simulink model "threepost_sim"  (R2020a)
settings: Solver=ode15s  StartTime=0.0  StopTime=T  FixedStep=0.00005  MaxStep=0.0005  RelTol=1e-3  EnableMultiTasking=on
values from neighbouring files (symbols this model uses):
  I_sat = [1/12*m_sat*(3*r^2+h^2),0,0;0,1/12*m_sat*(3*r^2+h^2),0;0,0,1/2*m_sat*r^2]    [berthing_sim_example_run.m]
  kd = 0.00005*[1;1;1;1;1;1;1]    [berthing_sim_example_run.m]
  ki = 0.001*ones(7,1)    [berthing_sim_example_run.m]
  kp = 5*[1;1;1;1;1;1;1]    [berthing_sim_example_run.m]
  m_sat = 2200    [berthing_sim_example_run.m]
  Pd = PBT0    [berthing_sim_example_run.m]
  q0 = [-0.0572;0.8617;0;-1.2870;0.0002;0.4292;0.0570]    [berthing_sim_example_run.m]
  qdot0 = zeros(7,1)    [berthing_sim_example_run.m]
  qlimit = [robot_const(1).limit.lower_joint_limit,     robot_const(1).limit.upper_joint_limit]    [berthing_sim_example_run.m]
  qm0 = robot_const.mprops.N.*q0    [berthing_sim_example_run.m]
  qmdot0 = zeros(7,1)    [berthing_sim_example_run.m]
  r = 0.7    [berthing_sim_example_run.m]
  ts_control = 0.002    [berthing_sim_example_run.m]
undefined symbols (not defined in the file or in its folder): robot_const, rot, X, Y, Z
libraries: sm_lib x58, nesl_utility x40, simulink x7
(part 1 of 3)
settings Model: Creator=Restore  LastModifiedBy=davidcarabis
settings SolverCC: MaxOrder=1  AutoInsertRateTranBlk=on
settings DataIOCC: ReturnWorkspaceOutputs=off
settings OptimizationCC: LifeSpan=inf
settings DebuggingCC: AllowSymbolicDim=off  SFUnexpectedBacktrackingDiag=warning  SFNoUnconditionalDefaultTransitionDiag=warning  SFExecutionAtInitializationDiag=none  ArithmeticOperatorsInVariantConditions=warning
settings SFSimCC: SimUseLocalCustomCode=off  CustomCodeUndefinedFunction=UseInterfaceOnly
settings RTWCC: RTWUseLocalCustomCode=off
settings CodeAppCC: StateflowObjectComments=on
settings GRTTargetCC: TargetLangStandard=C89/C90 (ANSI)
settings ConfigComp: CovMetricSettings=dw  CovHtmlReporting=on  CovSaveCumulativeToWorkspaceVar=on  CovSaveSingleToWorkspaceVar=on  CovExternalEMLEnable=off  CovSFcnEnable=off
settings SimscapeCC: SimscapeNominalValues="[{\"value\":\"10\",\"unit\":\"V\"},{\"value\":\"1\",\"unit\":\"A\"},{\"value\":\"10\",\"unit\":\"N*m\"},{\"value\":\"10\",\"unit\":\"bar\"},{\"value\":\"100\",\"unit\":\"kJ/kg\"},{\"value\":\"1\",\"unit\":\"kW\"},{\"value\":\"300\",\"unit\":\"K\"},{\"value\":\"100\",\"unit\":\"cm^3/s\"},{\"value\":\"1\",\"unit\":\"kN\"},{\"value\":\"1\",\"unit\":\"g/cm^3\"},{\"value\":\"1\",\"unit\":\"l\"},{\"value\":\"1\",\"unit\":\"cm^2\"},{\"value\":\"60\",\"unit\":\"Hz\"}]"  SimscapeLogType=all  SimscapeLogDataHistory=10000
settings ConfigurationSet: Description=SimMechanics 2G

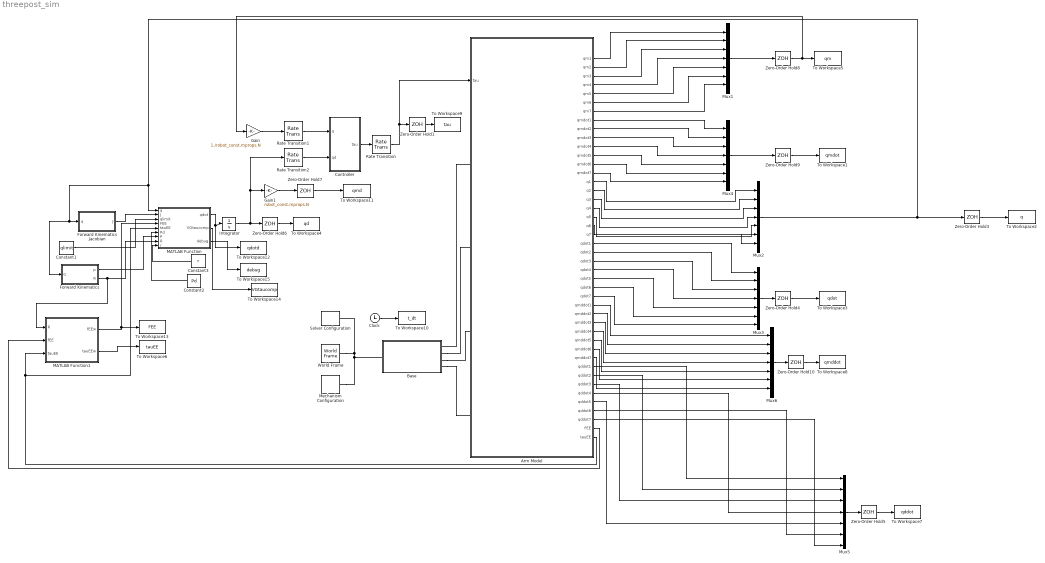
== system threepost_sim ==
  " Forward Kinematics Jacobian" : Subsystem  mask{H=robot_const(1).kin.H, P=robot_const.kin.P}
      mask prompts: H "Actuator Axes"; P "Actuator Displacements"
  Arm Model : Subsystem
  Base : Subsystem
  Clock : Clock
  Constant1 : Constant  Value=qlimit
  Constant2 : Constant  Value=Pd
  Constant3 : Constant  Value=r
  Controller : Subsystem
  Forward Kinematics : Subsystem  mask{H=robot_const(1).kin.H, P=robot_const(1).kin.P}
      mask prompts: H "Actuator Axes"; P "Actuator Displacements"
  Gain : Gain  Gain=1./robot_const.mprops.N
  Gain1 : Gain  Gain=robot_const.mprops.N
  Integrator : Integrator  InitialCondition=q0
  MATLAB Function : MATLAB Function  TreatAsAtomicUnit=on
  MATLAB Function1 : MATLAB Function  TreatAsAtomicUnit=on
  Mechanism Configuration : sm_lib/Utilities/Mechanism Configuration  UniformGravity=None  GravityVector=[0 0 -9.80665]  GravityUnits=m/s^2  LinearizationDelta=0.001
  Mux{1..6} (6 alike) : Mux  Inputs=7
  Rate Transition : RateTransition
  Rate Transition1 : RateTransition
  Rate Transition2 : RateTransition
  Solver Configuration : nesl_utility/Solver Configuration  PhysicalDomain=network_engine_domain  SubClassName=solver  LeftPortType=input  RightPortType=generic  Tones=[]  Harmonics=[]  SimulateNoise=off  Profile=off  UseLocalSampling=off  EnableSwitchedLinearOptims=on  FrequencyDomain=off  UseCCode=off  RelTol=0.001  AbsTol=1e-06  MinStep=1e-09  ToWorkspace=off  RevertToSquareIcSolve=off  NumHomotopyIterations=100  PhasorMode=off  PhasorModeNumHarmonics=1  DoDC=off  ResidualTolerance=1e-09  UseLocalSolver=off  LocalSolverChoice=NE_BACKWARD_EULER_ADVANCER  LocalSolverSampleTime=0.001  DoFixedCost=off  MaxNonlinIter=3  MaxModeIter=2  LinearAlgebra=Sparse  EquationFormulation=NE_TIME_EF  DelaysMemoryBudget=1024  AutomaticFiltering=on  FilteringTimeConstant=0.001  PartitionStorageMethod=AS_NEEDED  PartitionMemoryBudget=1024  PartitionMethod=FAST
  To Workspace1 : ToWorkspace  VariableName=qmdot  SampleTime=ts_control
  To Workspace10 : ToWorkspace  VariableName=t_dt  SampleTime=ts_control
  To Workspace11 : ToWorkspace  VariableName=qmd  SampleTime=-1
  To Workspace12 : ToWorkspace  VariableName=qdotd  SampleTime=-1
  To Workspace13 : ToWorkspace  VariableName=FEE  SampleTime=ts_control
  To Workspace14 : ToWorkspace  VariableName=VGtaucomp  SampleTime=-1
  To Workspace15 : ToWorkspace  VariableName=debug  SampleTime=-1
  To Workspace2 : ToWorkspace  VariableName=q  SampleTime=-1
  To Workspace3 : ToWorkspace  VariableName=qdot  SampleTime=-1
  To Workspace4 : ToWorkspace  VariableName=qd  SampleTime=-1
  To Workspace5 : ToWorkspace  VariableName=qm  SampleTime=ts_control
  To Workspace6 : ToWorkspace  VariableName=tauEE  SampleTime=ts_control
  To Workspace7 : ToWorkspace  VariableName=qddot  SampleTime=-1
  To Workspace8 : ToWorkspace  VariableName=qmddot  SampleTime=ts_control
  To Workspace9 : ToWorkspace  VariableName=tau  SampleTime=-1
  World Frame : sm_lib/Frames and Transforms/World Frame
  Zero-Order Hold{1,3..10} (9 alike) : ZeroOrderHold  SampleTime=ts_control
  wires:
  Arm Model/15(q1) -> Mux2/1
  Arm Model/16(q2) -> Mux2/2
  Arm Model/22(qdot1) -> Mux3/1
  Arm Model/23(qdot2) -> Mux3/2
  Mux3/1 -> Zero-Order Hold4/1
  Arm Model/17(q3) -> Mux2/3
  Arm Model/24(qdot3) -> Mux3/3
  Arm Model/18(q4) -> Mux2/4
  Arm Model/25(qdot4) -> Mux3/4
  Arm Model/19(q5) -> Mux2/5
  Arm Model/26(qdot5) -> Mux3/5
  Arm Model/20(q6) -> Mux2/6
  Arm Model/27(qdot6) -> Mux3/6
  Arm Model/21(q7) -> Mux2/7
  Arm Model/28(qdot7) -> Mux3/7
  Mux2/1 -> " Forward Kinematics Jacobian"/1(q), Forward Kinematics/1(q), MATLAB Function/1(q), Zero-Order Hold3/1
  Arm Model/36(qddot1) -> Mux5/1
  Arm Model/37(qddot2) -> Mux5/2
  Arm Model/38(qddot3) -> Mux5/3
  Mux5/1 -> Zero-Order Hold5/1
  Arm Model/39(qddot4) -> Mux5/4
  Arm Model/40(qddot5) -> Mux5/5
  Arm Model/41(qddot6) -> Mux5/6
  Arm Model/42(qddot7) -> Mux5/7
  Integrator/1 -> Gain1/1, Rate Transition2/1, Zero-Order Hold6/1
  Clock/1 -> To Workspace10/1
  Zero-Order Hold3/1 -> To Workspace2/1
  Zero-Order Hold4/1 -> To Workspace3/1
  Zero-Order Hold5/1 -> To Workspace7/1
  Zero-Order Hold6/1 -> To Workspace4/1
  Arm Model/1(qm1) -> Mux1/1
  Arm Model/2(qm2) -> Mux1/2
  Arm Model/3(qm3) -> Mux1/3
  Arm Model/4(qm4) -> Mux1/4
  Arm Model/5(qm5) -> Mux1/5
  Arm Model/6(qm6) -> Mux1/6
  Arm Model/7(qm7) -> Mux1/7
  Arm Model/8(qmdot1) -> Mux4/1
  Arm Model/9(qmdot2) -> Mux4/2
  Arm Model/10(qmdot3) -> Mux4/3
  Arm Model/11(qmdot4) -> Mux4/4
  Arm Model/12(qmdot5) -> Mux4/5
  Arm Model/13(qmdot6) -> Mux4/6
  Arm Model/14(qmdot7) -> Mux4/7
  Arm Model/29(qmddot1) -> Mux6/1
  Arm Model/30(qmddot2) -> Mux6/2
  Arm Model/31(qmddot3) -> Mux6/3
  Arm Model/32(qmddot4) -> Mux6/4
  Arm Model/33(qmddot5) -> Mux6/5
  Arm Model/34(qmddot6) -> Mux6/6
  Arm Model/35(qmddot7) -> Mux6/7
  Mux1/1 -> Zero-Order Hold8/1
  Mux4/1 -> Zero-Order Hold9/1
  Mux6/1 -> Zero-Order Hold10/1
  Zero-Order Hold9/1 -> To Workspace1/1
  Zero-Order Hold10/1 -> To Workspace8/1
  Zero-Order Hold8/1 -> Gain/1, To Workspace5/1
  Controller/1(tau) -> Rate Transition/1
  Rate Transition1/1 -> Controller/1(q)
  Rate Transition2/1 -> Controller/2(qd)
  Zero-Order Hold1/1 -> To Workspace9/1
  Gain/1 -> Rate Transition1/1
  Gain1/1 -> Zero-Order Hold7/1
  Zero-Order Hold7/1 -> To Workspace11/1
  Rate Transition/1 -> Zero-Order Hold1/1, Arm Model/1(tau)
  MATLAB Function/1(qdot) -> To Workspace12/1, Integrator/1
  " Forward Kinematics Jacobian"/1(J) -> MATLAB Function/2(J)
  Constant1/1 -> MATLAB Function/3(qlimit)
  Constant2/1 -> MATLAB Function/6(Pd)
  Forward Kinematics/2(R) -> MATLAB Function1/1(R), MATLAB Function/8(R)
  Forward Kinematics/1(p) -> MATLAB Function/7(P)
  MATLAB Function1/2(tauEEw) -> To Workspace6/1
  MATLAB Function1/1(fEEw) -> MATLAB Function/4(FEE), To Workspace13/1
  Arm Model/43(FEE) -> MATLAB Function1/2(fEE)
  Arm Model/44(tauEE) -> MATLAB Function/5(tauEE), MATLAB Function1/3(tauEE)
  Constant3/1 -> MATLAB Function/9(r)
  MATLAB Function/2(VGtaucomp) -> To Workspace14/1
  MATLAB Function/3(debug) -> To Workspace15/1
  connections:
  Mechanism Configuration/RConn1 -- Solver Configuration/RConn1 -- World Frame/RConn1 -- Base/LConn1
  Arm Model/LConn1 -- Base/RConn1
  Base/RConn2 -- Arm Model/LConn2
  Base/RConn3 -- Arm Model/LConn3
  Base/RConn4 -- Arm Model/LConn4

== system threepost_sim/ Forward Kinematics Jacobian ==
  q : Inport
  Forward Kinematics Jacobian : MATLAB Function  TreatAsAtomicUnit=on
  J : Outport
  wires:
  q/1 -> Forward Kinematics Jacobian/1(q)
  Forward Kinematics Jacobian/1(J) -> J/1

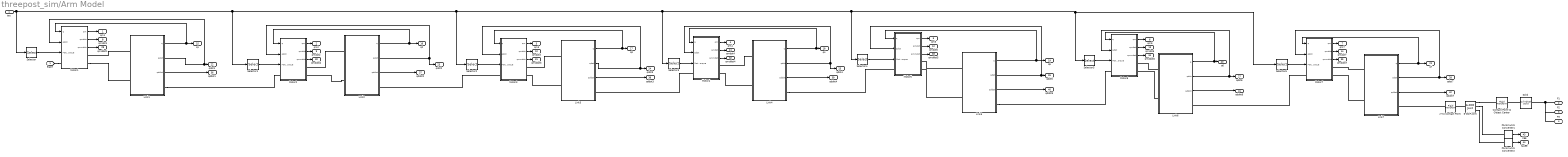
== system threepost_sim/Arm Model ==
  tau : Inport
  6-DOF Joint : sm_lib/Joints/6-DOF Joint  JointMode=Normal  SenseConstraintForce=off  SenseConstraintForceX=off  SenseConstraintForceY=off  SenseConstraintForceZ=off  SenseConstraintTorque=off  SenseConstraintTorqueX=off  SenseConstraintTorqueY=off  SenseConstraintTorqueZ=off  SenseTotalForce=on  SenseTotalForceX=off  SenseTotalForceY=off  SenseTotalForceZ=off  SenseTotalTorque=on  SenseTotalTorqueX=off  SenseTotalTorqueY=off  SenseTotalTorqueZ=off  CompositeWrenchDir=BaseOnFollower  CompositeWrenchFrame=BaseFrame  PxEquilibriumPosition=0  PxEquilibriumPositionUnits=m  PxSpringStiffness=kt_contact  PxSpringStiffnessUnits=N/m  PxDampingCoefficient=bt_contact  PxDampingCoefficientUnits=N/(m/s)  PxTorqueActuationMode=NoTorque  PxMotionActuationMode=ComputedMotion  PxSensePosition=off  PxSenseVelocity=off  PxSenseAcceleration=off  PxSenseTorqueForce=off  PxSenseLowerLimitTorqueForce=off  PxSenseUpperLimitTorqueForce=off  PxLowerLimitSpecify=off  PxLowerLimitBound=-1  PxLowerLimitBoundUnits=m  PxLowerLimitStiffness=1e6  PxLowerLimitStiffnessUnits=N/m  PxLowerLimitDamping=1e3  PxLowerLimitDampingUnits=N/(m/s)  PxLowerLimitTransitionRegionWidth=1e-4  PxLowerLimitTransitionRegionWidthUnits=m  PxUpperLimitSpecify=off  PxUpperLimitBound=1  PxUpperLimitBoundUnits=m  PxUpperLimitStiffness=1e6  PxUpperLimitStiffnessUnits=N/m  PxUpperLimitDamping=1e3  PxUpperLimitDampingUnits=N/(m/s)  PxUpperLimitTransitionRegionWidth=1e-4  PxUpperLimitTransitionRegionWidthUnits=m  PxPositionTargetSpecify=on  PxPositionTargetPriority=High  PxPositionTargetValue=0  PxPositionTargetValueUnits=m  PxVelocityTargetSpecify=on  PxVelocityTargetPriority=High  PxVelocityTargetValue=0  PxVelocityTargetValueUnits=m/s  PyEquilibriumPosition=0  PyEquilibriumPositionUnits=m  PySpringStiffness=kt_contact  PySpringStiffnessUnits=N/m  PyDampingCoefficient=bt_contact  PyDampingCoefficientUnits=N/(m/s)  PyTorqueActuationMode=NoTorque  PyMotionActuationMode=ComputedMotion  PySensePosition=off  PySenseVelocity=off  PySenseAcceleration=off  PySenseTorqueForce=off  PySenseLowerLimitTorqueForce=off  PySenseUpperLimitTorqueForce=off  PyLowerLimitSpecify=off  PyLowerLimitBound=-1  PyLowerLimitBoundUnits=m  PyLowerLimitStiffness=1e6  PyLowerLimitStiffnessUnits=N/m  PyLowerLimitDamping=1e3  PyLowerLimitDampingUnits=N/(m/s)  PyLowerLimitTransitionRegionWidth=1e-4  PyLowerLimitTransitionRegionWidthUnits=m  PyUpperLimitSpecify=off  PyUpperLimitBound=1  PyUpperLimitBoundUnits=m  PyUpperLimitStiffness=1e6  PyUpperLimitStiffnessUnits=N/m  PyUpperLimitDamping=1e3  PyUpperLimitDampingUnits=N/(m/s)  PyUpperLimitTransitionRegionWidth=1e-4  PyUpperLimitTransitionRegionWidthUnits=m  PyPositionTargetSpecify=on  PyPositionTargetPriority=High  PyPositionTargetValue=0  PyPositionTargetValueUnits=m  PyVelocityTargetSpecify=on  PyVelocityTargetPriority=High  PyVelocityTargetValue=0  PyVelocityTargetValueUnits=m/s  PzEquilibriumPosition=0  PzEquilibriumPositionUnits=m  PzSpringStiffness=kt_contact  PzSpringStiffnessUnits=N/m  PzDampingCoefficient=bt_contact  PzDampingCoefficientUnits=N/(m/s)  PzTorqueActuationMode=NoTorque  PzMotionActuationMode=ComputedMotion  PzSensePosition=off  PzSenseVelocity=off  PzSenseAcceleration=off  PzSenseTorqueForce=off  PzSenseLowerLimitTorqueForce=off  PzSenseUpperLimitTorqueForce=off  PzLowerLimitSpecify=off  PzLowerLimitBound=-1  PzLowerLimitBoundUnits=m  PzLowerLimitStiffness=1e6  PzLowerLimitStiffnessUnits=N/m  PzLowerLimitDamping=1e3  PzLowerLimitDampingUnits=N/(m/s)  PzLowerLimitTransitionRegionWidth=1e-4  PzLowerLimitTransitionRegionWidthUnits=m  PzUpperLimitSpecify=off  PzUpperLimitBound=1  PzUpperLimitBoundUnits=m  PzUpperLimitStiffness=1e6  PzUpperLimitStiffnessUnits=N/m  PzUpperLimitDamping=1e3  PzUpperLimitDampingUnits=N/(m/s)  PzUpperLimitTransitionRegionWidth=1e-4  PzUpperLimitTransitionRegionWidthUnits=m  PzPositionTargetSpecify=on  PzPositionTargetPriority=High  PzPositionTargetValue=0  PzPositionTargetValueUnits=m  PzVelocityTargetSpecify=on  PzVelocityTargetPriority=High  PzVelocityTargetValue=0  PzVelocityTargetValueUnits=m/s  SphDefPosRotationMethod=None  SphDefPosRotationAngleUnits=deg  SphDefPosRotationStandardAxis=+Z  SphDefPosRotationAngle=0.0  SphDefPosRotationArbitraryAxis=[0 0 1]  SphDefPosFollAlignAxisA=+X  SphDefPosBaseAlignAxisA=+Y  SphDefPosFollAlignAxisB=+Y  SphDefPosBaseAlignAxisB=+Z  SphDefPosRotationSequenceAxes=FollowerAxes  SphDefPosRotationSequence=XYX  SphDefPosRotationSequenceAngles=[0 0 0]  SphDefPosRotationSequenceAnglesUnits=deg  SphDefPosRotationMatrix=[1 0 0; 0 1 0; 0 0 1]  SphEqPosRotationMethod=RotationMatrix  SphEqPosRotationAngleUnits=deg  SphEqPosRotationStandardAxis=+Z  SphEqPosRotationAngle=0.0  SphEqPosRotationArbitraryAxis=[0 0 1]  SphEqPosFollAlignAxisA=+X  SphEqPosBaseAlignAxisA=+Y  SphEqPosFollAlignAxisB=+Y  SphEqPosBaseAlignAxisB=+Z  SphEqPosRotationSequenceAxes=FollowerAxes  SphEqPosRotationSequence=XYX  SphEqPosRotationSequenceAngles=[0 0 0]  SphEqPosRotationSequenceAnglesUnits=deg  SphEqPosRotationMatrix=[1 0 0; 0 1 0; 0 0 1]  SphSpringStiffness=kr_contact  SphSpringStiffnessUnits=N*m/rad  SphDampingCoefficient=br_contact  SphDampingCoefficientUnits=N*m/(rad/s)  SphActuateTorqueX=off  SphActuateTorqueY=off  SphActuateTorqueZ=off  SphActuateTorque=off  SphTorqueActuationMode=NoTorque  SphMotionActuationMode=ComputedMotion  SphActuationFrame=BaseFrame  SphSensePosition=off  SphSenseVelocityX=off  SphSenseVelocityY=off  SphSenseVelocityZ=off  SphSenseVelocity=off  SphSenseAccelerationX=off  SphSenseAccelerationY=off  SphSenseAccelerationZ=off  SphSenseAcceleration=off  SphSenseTorqueX=off  SphSenseTorqueY=off  SphSenseTorqueZ=off  SphSenseTorqueForce=off  SphSenseLowerLimitTorqueMag=off  SphSenseUpperLimitTorqueMag=off  SphSensingFrame=BaseFrame  SphLowerLimitSpecify=off  SphLowerLimitBound=15  SphLowerLimitBoundUnits=deg  SphLowerLimitStiffness=1e4  SphLowerLimitStiffnessUnits=N*m/deg  SphLowerLimitDamping=10  SphLowerLimitDampingUnits=N*m/(deg/s)  SphLowerLimitTransitionRegionWidth=0.1  SphLowerLimitTransitionRegionWidthUnits=deg  SphUpperLimitSpecify=off  SphUpperLimitBound=45  SphUpperLimitBoundUnits=deg  SphUpperLimitStiffness=1e4  SphUpperLimitStiffnessUnits=N*m/deg  SphUpperLimitDamping=10  SphUpperLimitDampingUnits=N*m/(deg/s)  SphUpperLimitTransitionRegionWidth=0.1  SphUpperLimitTransitionRegionWidthUnits=deg  SphPositionTargetRotationMethod=RotationMatrix  SphPositionTargetRotationAngleUnits=deg  SphPositionTargetRotationStandardAxis=+Z  SphPositionTargetRotationAngle=0.0  SphPositionTargetRotationArbitraryAxis=[0 0 1]  SphPositionTargetFollAlignAxisA=+X  SphPositionTargetBaseAlignAxisA=+Y  SphPositionTargetFollAlignAxisB=+Y  SphPositionTargetBaseAlignAxisB=+Z  SphPositionTargetRotationSequenceAxes=FollowerAxes  SphPositionTargetRotationSequence=XYX  SphPositionTargetRotationSequenceAngles=[0 0 0]  SphPositionTargetRotationSequenceAnglesUnits=deg  SphPositionTargetRotationMatrix=[1 0 0; 0 1 0; 0 0 1]  SphPositionTargetSpecify=on  SphPositionTargetPriority=High  SphVelocityTargetValue=[0 0 0]  SphVelocityTargetValueUnits=deg/s  SphVelocityTargetSpecify=on  SphVelocityTargetPriority=High  SphVelocityTargetInFollowerFrame=on
  Contact Point to Object Center : sm_lib/Frames and Transforms/Rigid Transform  TranslationMethod=Cartesian  TranslationStandardOffset=0  TranslationLengthUnit=m  TranslationStandardAxis=+Z  TranslationCartesianOffset=PGsat  TranslationROffset=0  TranslationROffsetUnits=m  TranslationZOffset=0  TranslationZOffsetUnits=m  TranslationThetaOffset=0  TranslationThetaOffsetUnits=deg  RotationMethod=None  RotationAngleUnits=rad  RotationStandardAxis=+Z  RotationAngle=0  RotationArbitraryAxis=0  FollAlignAxisA=+X  BaseAlignAxisA=+Y  FollAlignAxisB=+Y  BaseAlignAxisB=+Z  RotationSequenceAxes=FollowerAxes  RotationSequence=XYX  RotationSequenceAngles=[0 0 0]  RotationSequenceAnglesUnits=deg  RotationMatrix=[1 0 0; 0 1 0; 0 0 1]
  J7 to Contact Point : sm_lib/Frames and Transforms/Rigid Transform  TranslationMethod=Cartesian  TranslationStandardOffset=0  TranslationLengthUnit=m  TranslationStandardAxis=+Z  TranslationCartesianOffset=robot_const.kin.P(:,8)  TranslationROffset=0  TranslationROffsetUnits=m  TranslationZOffset=0  TranslationZOffsetUnits=m  TranslationThetaOffset=0  TranslationThetaOffsetUnits=deg  RotationMethod=None  RotationAngleUnits=rad  RotationStandardAxis=+Z  RotationAngle=0  RotationArbitraryAxis=0  FollAlignAxisA=+X  BaseAlignAxisA=+Y  FollAlignAxisB=+Y  BaseAlignAxisB=+Z  RotationSequenceAxes=FollowerAxes  RotationSequence=XYX  RotationSequenceAngles=[0 0 0]  RotationSequenceAnglesUnits=deg  RotationMatrix=[1 0 0; 0 1 0; 0 0 1]
  Link1 : Subsystem  mask{q0=q0(1), qdot0=qdot0(1), r=0.1, l=0.27035, m=robot_const.mprops.m(1), I=robot_const.mprops.Ic(:,:,1), c=robot_const.mprops.c(:,1), p=[0;0;0.27035/2]}
      mask prompts: q0 "Initial Position (rad)"; qdot0 "Initial Speed (rad/s)"; r "Radius (m)"; l "Length (m)"; m "Mass (kg)"; I "Inertia Tensor (kg m^2)"; c "COG Vector (m)"; p "Link Frame Translation"
  Link2 : Subsystem  mask{q0=q0(2), qdot0=qdot0(2), r=0.1, l=0.2, m=robot_const.mprops.m(2), I=[1 0 0;0 0 1 ;0 1 0]*robot_const.mprops.Ic(:,:,2)*[1 0 0;0 0 1 ;0 1 0]', c=[1 0 0;0 0 1 ;0 1 0]*robot_const.mprops.c(:,2), p=[0;0;0]}
      mask prompts: q0 "Initial Position (rad)"; qdot0 "Initial Speed (rad/s)"; r "Radius (m)"; l "Length (m)"; m "Mass (kg)"; I "Inertia Tensor (kg m^2)"; c "COG Vector (m)"; p "Link Frame Translation"
  Link3 : Subsystem  mask{q0=q0(3), qdot0=qdot0(3), r=0.08, l=0.36435, m=robot_const.mprops.m(3), I=robot_const.mprops.Ic(:,:,3), c=robot_const.mprops.c(:,3), p=[0;0;0.36435/2]}
      mask prompts: q0 "Initial Position (rad)"; qdot0 "Initial Speed (rad/s)"; r "Radius (m)"; l "Length (m)"; m "Mass (kg)"; I "Inertia Tensor (kg m^2)"; c "COG Vector (m)"; p "Link Frame Translation"
  Link4 : Subsystem  mask{q0=q0(4), qdot0=qdot0(4), r=0.08, l=0.2, m=robot_const.mprops.m(4), I=[1 0 0;0 0 1 ;0 1 0]*robot_const.mprops.Ic(:,:,4)*[1 0 0;0 0 1 ;0 1 0]', c=[1 0 0;0 0 1 ;0 1 0]*robot_const.mprops.c(:,4), p=[0;0;0]}
      mask prompts: q0 "Initial Position (rad)"; qdot0 "Initial Speed (rad/s)"; r "Radius (m)"; l "Length (m)"; m "Mass (kg)"; I "Inertia Tensor (kg m^2)"; c "COG Vector (m)"; p "Link Frame Translation"
  Link5 : Subsystem  mask{q0=q0(5), qdot0=qdot0(5), r=0.08, l=0.37429, m=robot_const.mprops.m(5), I=robot_const.mprops.Ic(:,:,5), c=robot_const.mprops.c(:,5), p=[0;0;0.37429/2]}
      mask prompts: q0 "Initial Position (rad)"; qdot0 "Initial Speed (rad/s)"; r "Radius (m)"; l "Length (m)"; m "Mass (kg)"; I "Inertia Tensor (kg m^2)"; c "COG Vector (m)"; p "Link Frame Translation"
  Link6 : Subsystem  mask{q0=q0(6), qdot0=qdot0(6), r=0.08, l=0.2, m=robot_const.mprops.m(6), I=[1 0 0;0 0 1 ;0 1 0]*robot_const.mprops.Ic(:,:,6)*[1 0 0;0 0 1 ;0 1 0]', c=[1 0 0;0 0 1 ;0 1 0]*robot_const.mprops.c(:,6), p=[0;0;0]}
      mask prompts: q0 "Initial Position (rad)"; qdot0 "Initial Speed (rad/s)"; r "Radius (m)"; l "Length (m)"; m "Mass (kg)"; I "Inertia Tensor (kg m^2)"; c "COG Vector (m)"; p "Link Frame Translation"
  Link7 : Subsystem  mask{q0=q0(7), qdot0=qdot0(7), r=0.05, l=robot_const.kin.P(3,8), m=robot_const.mprops.m(7), I=robot_const.mprops.Ic(:,:,7), c=robot_const.mprops.c(:,7), p=robot_const.kin.P(:,8)/2}
      mask prompts: q0 "Initial Position (rad)"; qdot0 "Initial Speed (rad/s)"; r "Radius (m)"; l "Length (m)"; m "Mass (kg)"; I "Inertia Tensor (kg m^2)"; c "COG Vector (m)"; p "Link Frame Translation"
  Motor1 : Subsystem  mask{h=[1;0;0], alpha=0, p=[0;0;0], bm=robot_const.mprops.bm(1), Jm=robot_const.mprops.Im(1), N=robot_const.mprops.N(1), K=robot_const.mprops.K(1), bL=robot_const.mprops.bl(1), qm0=qm0(1), qmdot0=qmdot0(1)}
      mask prompts: h "Frame Rotation Axis"; alpha "Frame Rotation Angle (rad)"; p "Frame Translation (m)"; bm "Motor Friction"; Jm "Motor Inertia (kg m^2)"; N "Gear Ratio"; K "Spring Constant (Nm/rad)"; bL "Gearbox Friction (Nm s/rad)"; qm0 "Motor Initial Position"; qmdot0 "Motor Initial Velocity"
  Motor2 : Subsystem  mask{h=[1;0;0], alpha=-pi/2, p=robot_const.kin.P(:,2), bm=robot_const.mprops.bm(2), Jm=robot_const.mprops.Im(2), N=robot_const.mprops.N(2), K=robot_const.mprops.K(2), bL=robot_const.mprops.bl(2), qm0=qm0(2), qmdot0=qmdot0(2)}
      mask prompts: h "Frame Rotation Axis"; alpha "Frame Rotation Angle (rad)"; p "Frame Translation (m)"; bm "Motor Friction"; Jm "Motor Inertia (kg m^2)"; N "Gear Ratio"; K "Spring Constant (Nm/rad)"; bL "Gearbox Friction (Nm s/rad)"; qm0 "Motor Initial Position"; qmdot0 "Motor Initial Velocity"
  Motor3 : Subsystem  mask{h=[1;0;0], alpha=0, p=[0;0;0], bm=robot_const.mprops.bm(3), Jm=robot_const.mprops.Im(3), N=robot_const.mprops.N(3), K=robot_const.mprops.K(3), bL=robot_const.mprops.bl(3), qm0=qm0(3), qmdot0=qmdot0(3)}
      mask prompts: h "Frame Rotation Axis"; alpha "Frame Rotation Angle (rad)"; p "Frame Translation (m)"; bm "Motor Friction"; Jm "Motor Inertia (kg m^2)"; N "Gear Ratio"; K "Spring Constant (Nm/rad)"; bL "Gearbox Friction (Nm s/rad)"; qm0 "Motor Initial Position"; qmdot0 "Motor Initial Velocity"
  Motor4 : Subsystem  mask{h=[1;0;0], alpha=-pi/2, p=robot_const.kin.P(:,4), bm=robot_const.mprops.bm(4), Jm=robot_const.mprops.Im(4), N=robot_const.mprops.N(4), K=robot_const.mprops.K(4), bL=robot_const.mprops.bl(4), qm0=qm0(4), qmdot0=qmdot0(4)}
      mask prompts: h "Frame Rotation Axis"; alpha "Frame Rotation Angle (rad)"; p "Frame Translation (m)"; bm "Motor Friction"; Jm "Motor Inertia (kg m^2)"; N "Gear Ratio"; K "Spring Constant (Nm/rad)"; bL "Gearbox Friction (Nm s/rad)"; qm0 "Motor Initial Position"; qmdot0 "Motor Initial Velocity"
  Motor5 : Subsystem  mask{h=[1;0;0], alpha=0, p=[0;0;0], bm=robot_const.mprops.bm(5), Jm=robot_const.mprops.Im(5), N=robot_const.mprops.N(5), K=robot_const.mprops.K(5), bL=robot_const.mprops.bl(5), qm0=qm0(5), qmdot0=qmdot0(5)}
      mask prompts: h "Frame Rotation Axis"; alpha "Frame Rotation Angle (rad)"; p "Frame Translation (m)"; bm "Motor Friction"; Jm "Motor Inertia (kg m^2)"; N "Gear Ratio"; K "Spring Constant (Nm/rad)"; bL "Gearbox Friction (Nm s/rad)"; qm0 "Motor Initial Position"; qmdot0 "Motor Initial Velocity"
  Motor6 : Subsystem  mask{h=[1;0;0], alpha=-pi/2, p=robot_const.kin.P(:,6), bm=robot_const.mprops.bm(6), Jm=robot_const.mprops.Im(6), N=robot_const.mprops.N(6), K=robot_const.mprops.K(6), bL=robot_const.mprops.bl(6), qm0=qm0(6), qmdot0=qmdot0(6)}
      mask prompts: h "Frame Rotation Axis"; alpha "Frame Rotation Angle (rad)"; p "Frame Translation (m)"; bm "Motor Friction"; Jm "Motor Inertia (kg m^2)"; N "Gear Ratio"; K "Spring Constant (Nm/rad)"; bL "Gearbox Friction (Nm s/rad)"; qm0 "Motor Initial Position"; qmdot0 "Motor Initial Velocity"
  Motor7 : Subsystem  mask{h=[1;0;0], alpha=0, p=[0;0;0], bm=robot_const.mprops.bm(7), Jm=robot_const.mprops.Im(7), N=robot_const.mprops.N(7), K=robot_const.mprops.K(7), bL=robot_const.mprops.bl(7), qm0=qm0(7), qmdot0=qmdot0(7)}
      mask prompts: h "Frame Rotation Axis"; alpha "Frame Rotation Angle (rad)"; p "Frame Translation (m)"; bm "Motor Friction"; Jm "Motor Inertia (kg m^2)"; N "Gear Ratio"; K "Spring Constant (Nm/rad)"; bL "Gearbox Friction (Nm s/rad)"; qm0 "Motor Initial Position"; qmdot0 "Motor Initial Velocity"
  PS-Simulink Converter1 : nesl_utility/PS-Simulink Converter  PhysicalDomain=network_engine_domain  SubClassName=ps_output  LeftPortType=input  RightPortType=output  PseudoPeriodic=off  Frequencies=[]  Unit=1  AffineConversion=off
  PS-Simulink Converter2 : nesl_utility/PS-Simulink Converter  PhysicalDomain=network_engine_domain  SubClassName=ps_output  LeftPortType=input  RightPortType=output  PseudoPeriodic=off  Frequencies=[]  Unit=1  AffineConversion=off
  Selector : Selector  InputPortWidth=7  IndexOptions=Index vector (dialog)  Indices=[1]  OutputSizes=1
  Selector1 : Selector  InputPortWidth=7  IndexOptions=Index vector (dialog)  Indices=[2]  OutputSizes=1
  Selector2 : Selector  InputPortWidth=7  IndexOptions=Index vector (dialog)  Indices=[3]  OutputSizes=1
  Selector3 : Selector  InputPortWidth=7  IndexOptions=Index vector (dialog)  Indices=[4]  OutputSizes=1
  Selector4 : Selector  InputPortWidth=7  IndexOptions=Index vector (dialog)  Indices=[5]  OutputSizes=1
  Selector5 : Selector  InputPortWidth=7  IndexOptions=Index vector (dialog)  Indices=[6]  OutputSizes=1
  Selector6 : Selector  InputPortWidth=7  IndexOptions=Index vector (dialog)  Indices=[7]  OutputSizes=1
  Solid : sm_lib/Body Elements/Cylindrical Solid  GraphicAmbientColor=[0.15 0.15 0.15 1.0]  BasedOnType=Density  CenterOfMass=c_sat  CenterOfMassUnits=m  GraphicDiffuseColor=[0.6 0.6 0.0]  CylinderLength=h  CylinderLengthUnits=m  CylinderRadius=r  CylinderRadiusUnits=m  Density=1000  DensityUnits=kg/m^3  DoExposeReferenceFrame=on  GraphicEmissiveColor=[0.0 0.0 0.0 1.0]  ExportEntireGeometry=on  SerializedFrames=<Frames/>  MarkerShape=Sphere  MarkerSize=10  GraphicType=FromGeometry  InertiaType=Custom  Mass=m_sat  MassUnits=kg  MomentsOfInertia=[I_sat(1,1) I_sat(2,2) I_sat(3,3)]  MomentsOfInertiaUnits=kg*m^2  GraphicOpacity=1.0  ProductsOfInertia=[I_sat(2,3) I_sat(3,1) I_sat(1,2)]  ProductsOfInertiaUnits=kg*m^2  GraphicShininess=75  GraphicSpecularColor=[0.5 0.5 0.5 1.0]  GraphicVisPropType=SimpleVisualProperties
  Base : PMIOPort  Side=Left
  P1 : PMIOPort  Port=2  Side=Left
  P2 : PMIOPort  Port=3  Side=Left
  P3 : PMIOPort  Port=4  Side=Left
  qm1 : Outport  VectorParamsAs1DForOutWhenUnconnected=off
  qm2 : Outport  Port=2  VectorParamsAs1DForOutWhenUnconnected=off
  qm3 : Outport  Port=3  VectorParamsAs1DForOutWhenUnconnected=off
  qm4 : Outport  Port=4  VectorParamsAs1DForOutWhenUnconnected=off
  qm5 : Outport  Port=5  VectorParamsAs1DForOutWhenUnconnected=off
  qm6 : Outport  Port=6  VectorParamsAs1DForOutWhenUnconnected=off
  qm7 : Outport  Port=7  VectorParamsAs1DForOutWhenUnconnected=off
  qmdot1 : Outport  Port=8  VectorParamsAs1DForOutWhenUnconnected=off
  qmdot2 : Outport  Port=9  VectorParamsAs1DForOutWhenUnconnected=off
  qmdot3 : Outport  Port=10  VectorParamsAs1DForOutWhenUnconnected=off
  qmdot4 : Outport  Port=11  VectorParamsAs1DForOutWhenUnconnected=off
  qmdot5 : Outport  Port=12  VectorParamsAs1DForOutWhenUnconnected=off
  qmdot6 : Outport  Port=13  VectorParamsAs1DForOutWhenUnconnected=off
  qmdot7 : Outport  Port=14  VectorParamsAs1DForOutWhenUnconnected=off
  q1 : Outport  Port=15  VectorParamsAs1DForOutWhenUnconnected=off
  q2 : Outport  Port=16  VectorParamsAs1DForOutWhenUnconnected=off
  q3 : Outport  Port=17  VectorParamsAs1DForOutWhenUnconnected=off
  q4 : Outport  Port=18  VectorParamsAs1DForOutWhenUnconnected=off
  q5 : Outport  Port=19  VectorParamsAs1DForOutWhenUnconnected=off
  q6 : Outport  Port=20  VectorParamsAs1DForOutWhenUnconnected=off
  q7 : Outport  Port=21  VectorParamsAs1DForOutWhenUnconnected=off
  qdot1 : Outport  Port=22  VectorParamsAs1DForOutWhenUnconnected=off
  qdot2 : Outport  Port=23  VectorParamsAs1DForOutWhenUnconnected=off
  qdot3 : Outport  Port=24  VectorParamsAs1DForOutWhenUnconnected=off
  qdot4 : Outport  Port=25  VectorParamsAs1DForOutWhenUnconnected=off
  qdot5 : Outport  Port=26  VectorParamsAs1DForOutWhenUnconnected=off
  qdot6 : Outport  Port=27  VectorParamsAs1DForOutWhenUnconnected=off
  qdot7 : Outport  Port=28  VectorParamsAs1DForOutWhenUnconnected=off
  qmddot1 : Outport  Port=29  VectorParamsAs1DForOutWhenUnconnected=off
  qmddot2 : Outport  Port=30  VectorParamsAs1DForOutWhenUnconnected=off
  qmddot3 : Outport  Port=31  VectorParamsAs1DForOutWhenUnconnected=off
  qmddot4 : Outport  Port=32  VectorParamsAs1DForOutWhenUnconnected=off
  qmddot5 : Outport  Port=33  VectorParamsAs1DForOutWhenUnconnected=off
  qmddot6 : Outport  Port=34  VectorParamsAs1DForOutWhenUnconnected=off
  qmddot7 : Outport  Port=35  VectorParamsAs1DForOutWhenUnconnected=off
  qddot1 : Outport  Port=36  VectorParamsAs1DForOutWhenUnconnected=off
  qddot2 : Outport  Port=37  VectorParamsAs1DForOutWhenUnconnected=off
  qddot3 : Outport  Port=38  VectorParamsAs1DForOutWhenUnconnected=off
  qddot4 : Outport  Port=39  VectorParamsAs1DForOutWhenUnconnected=off
  qddot5 : Outport  Port=40  VectorParamsAs1DForOutWhenUnconnected=off
  qddot6 : Outport  Port=41  VectorParamsAs1DForOutWhenUnconnected=off
  qddot7 : Outport  Port=42  VectorParamsAs1DForOutWhenUnconnected=off
  FEE : Outport  Port=43  VectorParamsAs1DForOutWhenUnconnected=off
  tauEE : Outport  Port=44  VectorParamsAs1DForOutWhenUnconnected=off
  wires:
  Selector1/1 -> Motor2/3(Motor Torque)
  Selector2/1 -> Motor3/3(Motor Torque)
  Selector/1 -> Motor1/3(Motor Torque)
  Selector3/1 -> Motor4/3(Motor Torque)
  Selector4/1 -> Motor5/3(Motor Torque)
  Selector5/1 -> Motor6/3(Motor Torque)
  Selector6/1 -> Motor7/3(Motor Torque)
  Link1/1(q) -> q1/1, Motor1/1(q)
  Link1/2(qdot) -> Motor1/2(qdot), qdot1/1
  Link1/3(qddot) -> qddot1/1
  Link2/1(q) -> Motor2/1(q), q2/1
  Link2/2(qdot) -> Motor2/2(qdot), qdot2/1
  Link2/3(qddot) -> qddot2/1
  Link3/1(q) -> Motor3/1(q), q3/1
  Link3/2(qdot) -> Motor3/2(qdot), qdot3/1
  Link3/3(qddot) -> qddot3/1
  Link4/1(q) -> Motor4/1(q), q4/1
  Link4/2(qdot) -> qdot4/1, Motor4/2(qdot)
  Link4/3(qddot) -> qddot4/1
  Link5/1(q) -> Motor5/1(q), q5/1
  Link5/2(qdot) -> Motor5/2(qdot), qdot5/1
  Link5/3(qddot) -> qddot5/1
  Link6/2(qdot) -> Motor6/2(qdot), qdot6/1
  Link6/1(q) -> Motor6/1(q), q6/1
  Link6/3(qddot) -> qddot6/1
  Link7/3(qddot) -> qddot7/1
  Link7/2(qdot) -> Motor7/2(qdot), qdot7/1
  Link7/1(q) -> Motor7/1(q), q7/1
  tau/1 -> Selector/1, Selector1/1, Selector3/1, Selector6/1, Selector5/1, Selector4/1, Selector2/1
  Motor1/3(qmmdot) -> qmddot1/1
  Motor1/2(qmdot) -> qmdot1/1
  Motor1/1(qm) -> qm1/1
  Motor2/1(qm) -> qm2/1
  Motor2/2(qmdot) -> qmdot2/1
  Motor2/3(qmmdot) -> qmddot2/1
  Motor3/1(qm) -> qm3/1
  Motor3/2(qmdot) -> qmdot3/1
  Motor3/3(qmmdot) -> qmddot3/1
  Motor4/1(qm) -> qm4/1
  Motor4/2(qmdot) -> qmdot4/1
  Motor4/3(qmmdot) -> qmddot4/1
  Motor5/1(qm) -> qm5/1
  Motor5/2(qmdot) -> qmdot5/1
  Motor5/3(qmmdot) -> qmddot5/1
  Motor6/1(qm) -> qm6/1
  Motor6/2(qmdot) -> qmdot6/1
  Motor6/3(qmmdot) -> qmddot6/1
  Motor7/1(qm) -> qm7/1
  Motor7/2(qmdot) -> qmdot7/1
  Motor7/3(qmmdot) -> qmddot7/1
  PS-Simulink Converter1/1 -> FEE/1
  PS-Simulink Converter2/1 -> tauEE/1
  connections:
  Base/RConn1 -- Motor1/LConn1
  Link1/RConn1 -- Motor2/LConn1
  Link3/LConn1 -- Motor3/RConn1
  Link1/LConn1 -- Motor1/RConn1
  Link2/LConn1 -- Motor2/RConn1
  Link3/LConn2 -- Motor3/RConn2
  Link2/LConn2 -- Motor2/RConn2
  Motor1/RConn2 -- Link1/LConn2
  Motor4/LConn1 -- Link3/RConn1
  Link4/LConn1 -- Motor4/RConn1
  Link4/LConn2 -- Motor4/RConn2
  Link4/RConn1 -- Motor5/LConn1
  Link5/LConn1 -- Motor5/RConn1
  Link5/LConn2 -- Motor5/RConn2
  Link5/RConn1 -- Motor6/LConn1
  Link6/LConn2 -- Motor6/RConn2
  Link6/LConn1 -- Motor6/RConn1
  Motor7/LConn1 -- Link6/RConn1
  Link7/LConn2 -- Motor7/RConn2
  Link7/LConn1 -- Motor7/RConn1
  J7 to Contact Point/LConn1 -- Link7/RConn1
  6-DOF Joint/LConn1 -- J7 to Contact Point/RConn1
  Solid/RConn1 -- Contact Point to Object Center/RConn1
  Motor3/LConn1 -- Link2/RConn1
  6-DOF Joint/RConn1 -- Contact Point to Object Center/LConn1
  6-DOF Joint/RConn2 -- PS-Simulink Converter1/LConn1
  6-DOF Joint/RConn3 -- PS-Simulink Converter2/LConn1
  P1/RConn1 -- P3/RConn1 -- P2/RConn1 -- Solid/LConn1

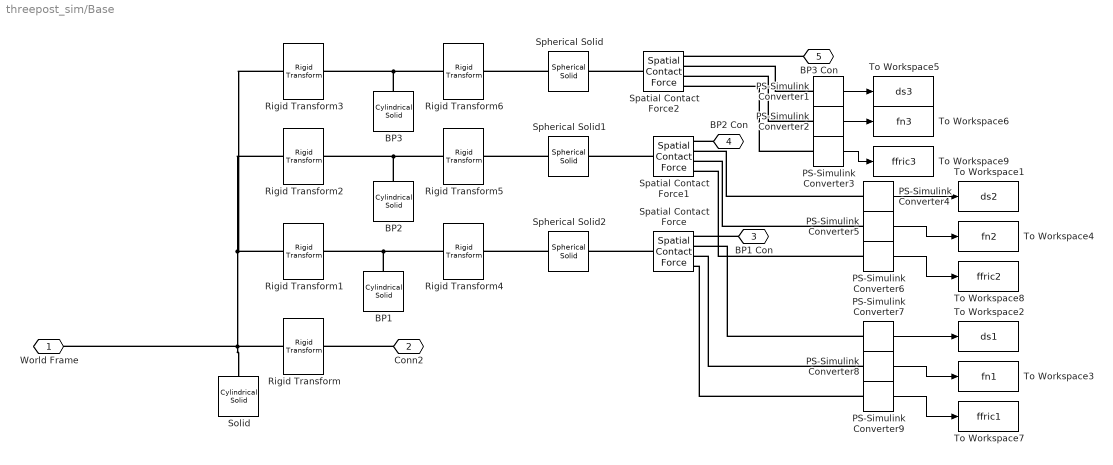
== system threepost_sim/Base ==
  BP1 : sm_lib/Body Elements/Cylindrical Solid  GraphicAmbientColor=[0.15 0.15 0.15 1.0]  BasedOnType=Density  CenterOfMass=[0 0 0]  CenterOfMassUnits=m  GraphicDiffuseColor=[0.4 0.4 0.4]  CylinderLength=1  CylinderLengthUnits=m  CylinderRadius=0.1  CylinderRadiusUnits=m  Density=1000  DensityUnits=kg/m^3  DoExposeReferenceFrame=on  GraphicEmissiveColor=[0.0 0.0 0.0 1.0]  ExportEntireGeometry=off  SerializedFrames=<Frames/>  MarkerShape=Sphere  MarkerSize=10  GraphicType=FromGeometry  InertiaType=CalculateFromGeometry  Mass=1  MassUnits=kg  MomentsOfInertia=[1 1 1]  MomentsOfInertiaUnits=kg*m^2  GraphicOpacity=1.0  ProductsOfInertia=[0 0 0]  ProductsOfInertiaUnits=kg*m^2  GraphicShininess=75  GraphicSpecularColor=[0.5 0.5 0.5 1.0]  GraphicVisPropType=SimpleVisualProperties
  BP2 : sm_lib/Body Elements/Cylindrical Solid  GraphicAmbientColor=[0.15 0.15 0.15 1.0]  BasedOnType=Density  CenterOfMass=[0 0 0]  CenterOfMassUnits=m  GraphicDiffuseColor=[0.4 0.4 0.4]  CylinderLength=1  CylinderLengthUnits=m  CylinderRadius=0.1  CylinderRadiusUnits=m  Density=1000  DensityUnits=kg/m^3  DoExposeReferenceFrame=on  GraphicEmissiveColor=[0.0 0.0 0.0 1.0]  ExportEntireGeometry=off  SerializedFrames=<Frames/>  MarkerShape=Sphere  MarkerSize=10  GraphicType=FromGeometry  InertiaType=CalculateFromGeometry  Mass=1  MassUnits=kg  MomentsOfInertia=[1 1 1]  MomentsOfInertiaUnits=kg*m^2  GraphicOpacity=1.0  ProductsOfInertia=[0 0 0]  ProductsOfInertiaUnits=kg*m^2  GraphicShininess=75  GraphicSpecularColor=[0.5 0.5 0.5 1.0]  GraphicVisPropType=SimpleVisualProperties
  BP3 : sm_lib/Body Elements/Cylindrical Solid  GraphicAmbientColor=[0.15 0.15 0.15 1.0]  BasedOnType=Density  CenterOfMass=[0 0 0]  CenterOfMassUnits=m  GraphicDiffuseColor=[0.4 0.4 0.4]  CylinderLength=1  CylinderLengthUnits=m  CylinderRadius=0.1  CylinderRadiusUnits=m  Density=1000  DensityUnits=kg/m^3  DoExposeReferenceFrame=on  GraphicEmissiveColor=[0.0 0.0 0.0 1.0]  ExportEntireGeometry=off  SerializedFrames=<Frames/>  MarkerShape=Sphere  MarkerSize=10  GraphicType=FromGeometry  InertiaType=CalculateFromGeometry  Mass=1  MassUnits=kg  MomentsOfInertia=[1 1 1]  MomentsOfInertiaUnits=kg*m^2  GraphicOpacity=1.0  ProductsOfInertia=[0 0 0]  ProductsOfInertiaUnits=kg*m^2  GraphicShininess=75  GraphicSpecularColor=[0.5 0.5 0.5 1.0]  GraphicVisPropType=SimpleVisualProperties
  PS-Simulink Converter{1..9} (9 alike) : nesl_utility/PS-Simulink Converter  PhysicalDomain=network_engine_domain  SubClassName=ps_output  LeftPortType=input  RightPortType=output  PseudoPeriodic=off  Frequencies=[]  Unit=1  AffineConversion=off
  Rigid Transform : sm_lib/Frames and Transforms/Rigid Transform  TranslationMethod=Cartesian  TranslationStandardOffset=0  TranslationLengthUnit=m  TranslationStandardAxis=+Z  TranslationCartesianOffset=[1;0;2.5]  TranslationROffset=0  TranslationROffsetUnits=m  TranslationZOffset=0  TranslationZOffsetUnits=m  TranslationThetaOffset=0  TranslationThetaOffsetUnits=deg  RotationMethod=None  RotationAngleUnits=rad  RotationStandardAxis=+Z  RotationAngle=0  RotationArbitraryAxis=[0;0;0]  FollAlignAxisA=+X  BaseAlignAxisA=+Y  FollAlignAxisB=+Y  BaseAlignAxisB=+Z  RotationSequenceAxes=FollowerAxes  RotationSequence=XYX  RotationSequenceAngles=[0 0 0]  RotationSequenceAnglesUnits=deg  RotationMatrix=[1 0 0; 0 1 0; 0 0 1]
  Rigid Transform1 : sm_lib/Frames and Transforms/Rigid Transform  TranslationMethod=Cartesian  TranslationStandardOffset=0  TranslationLengthUnit=m  TranslationStandardAxis=+Z  TranslationCartesianOffset=[1-1.8*r;0;3]  TranslationROffset=0  TranslationROffsetUnits=m  TranslationZOffset=0  TranslationZOffsetUnits=m  TranslationThetaOffset=0  TranslationThetaOffsetUnits=deg  RotationMethod=None  RotationAngleUnits=rad  RotationStandardAxis=+Z  RotationAngle=0  RotationArbitraryAxis=[0;0;0]  FollAlignAxisA=+X  BaseAlignAxisA=+Y  FollAlignAxisB=+Y  BaseAlignAxisB=+Z  RotationSequenceAxes=FollowerAxes  RotationSequence=XYX  RotationSequenceAngles=[0 0 0]  RotationSequenceAnglesUnits=deg  RotationMatrix=[1 0 0; 0 1 0; 0 0 1]
  Rigid Transform2 : sm_lib/Frames and Transforms/Rigid Transform  TranslationMethod=Cartesian  TranslationStandardOffset=0  TranslationLengthUnit=m  TranslationStandardAxis=+Z  TranslationCartesianOffset=[1-r;-0.8*r;3]  TranslationROffset=0  TranslationROffsetUnits=m  TranslationZOffset=0  TranslationZOffsetUnits=m  TranslationThetaOffset=0  TranslationThetaOffsetUnits=deg  RotationMethod=None  RotationAngleUnits=rad  RotationStandardAxis=+Z  RotationAngle=0  RotationArbitraryAxis=[0;0;0]  FollAlignAxisA=+X  BaseAlignAxisA=+Y  FollAlignAxisB=+Y  BaseAlignAxisB=+Z  RotationSequenceAxes=FollowerAxes  RotationSequence=XYX  RotationSequenceAngles=[0 0 0]  RotationSequenceAnglesUnits=deg  RotationMatrix=[1 0 0; 0 1 0; 0 0 1]
  Rigid Transform3 : sm_lib/Frames and Transforms/Rigid Transform  TranslationMethod=Cartesian  TranslationStandardOffset=0  TranslationLengthUnit=m  TranslationStandardAxis=+Z  TranslationCartesianOffset=[1-r;0.8*r;3]  TranslationROffset=0  TranslationROffsetUnits=m  TranslationZOffset=0  TranslationZOffsetUnits=m  TranslationThetaOffset=0  TranslationThetaOffsetUnits=deg  RotationMethod=None  RotationAngleUnits=rad  RotationStandardAxis=+Z  RotationAngle=0  RotationArbitraryAxis=[0;0;0]  FollAlignAxisA=+X  BaseAlignAxisA=+Y  FollAlignAxisB=+Y  BaseAlignAxisB=+Z  RotationSequenceAxes=FollowerAxes  RotationSequence=XYX  RotationSequenceAngles=[0 0 0]  RotationSequenceAnglesUnits=deg  RotationMatrix=[1 0 0; 0 1 0; 0 0 1]
  Rigid Transform4 : sm_lib/Frames and Transforms/Rigid Transform  TranslationMethod=Cartesian  TranslationStandardOffset=0  TranslationLengthUnit=m  TranslationStandardAxis=+Z  TranslationCartesianOffset=[0;0;0.5]  TranslationROffset=0  TranslationROffsetUnits=m  TranslationZOffset=0  TranslationZOffsetUnits=m  TranslationThetaOffset=0  TranslationThetaOffsetUnits=deg  RotationMethod=None  RotationAngleUnits=rad  RotationStandardAxis=+Z  RotationAngle=0  RotationArbitraryAxis=[0;0;0]  FollAlignAxisA=+X  BaseAlignAxisA=+Y  FollAlignAxisB=+Y  BaseAlignAxisB=+Z  RotationSequenceAxes=FollowerAxes  RotationSequence=XYX  RotationSequenceAngles=[0 0 0]  RotationSequenceAnglesUnits=deg  RotationMatrix=[1 0 0; 0 1 0; 0 0 1]
  Rigid Transform5 : sm_lib/Frames and Transforms/Rigid Transform  TranslationMethod=Cartesian  TranslationStandardOffset=0  TranslationLengthUnit=m  TranslationStandardAxis=+Z  TranslationCartesianOffset=[0;0;0.5]  TranslationROffset=0  TranslationROffsetUnits=m  TranslationZOffset=0  TranslationZOffsetUnits=m  TranslationThetaOffset=0  TranslationThetaOffsetUnits=deg  RotationMethod=None  RotationAngleUnits=rad  RotationStandardAxis=+Z  RotationAngle=0  RotationArbitraryAxis=[0;0;0]  FollAlignAxisA=+X  BaseAlignAxisA=+Y  FollAlignAxisB=+Y  BaseAlignAxisB=+Z  RotationSequenceAxes=FollowerAxes  RotationSequence=XYX  RotationSequenceAngles=[0 0 0]  RotationSequenceAnglesUnits=deg  RotationMatrix=[1 0 0; 0 1 0; 0 0 1]
  Rigid Transform6 : sm_lib/Frames and Transforms/Rigid Transform  TranslationMethod=Cartesian  TranslationStandardOffset=0  TranslationLengthUnit=m  TranslationStandardAxis=+Z  TranslationCartesianOffset=[0;0;0.5]  TranslationROffset=0  TranslationROffsetUnits=m  TranslationZOffset=0  TranslationZOffsetUnits=m  TranslationThetaOffset=0  TranslationThetaOffsetUnits=deg  RotationMethod=None  RotationAngleUnits=rad  RotationStandardAxis=+Z  RotationAngle=0  RotationArbitraryAxis=[0;0;0]  FollAlignAxisA=+X  BaseAlignAxisA=+Y  FollAlignAxisB=+Y  BaseAlignAxisB=+Z  RotationSequenceAxes=FollowerAxes  RotationSequence=XYX  RotationSequenceAngles=[0 0 0]  RotationSequenceAnglesUnits=deg  RotationMatrix=[1 0 0; 0 1 0; 0 0 1]
  Solid : sm_lib/Body Elements/Cylindrical Solid  GraphicAmbientColor=[0.15 0.15 0.15 1.0]  BasedOnType=Density  CenterOfMass=[0 0 0]  CenterOfMassUnits=m  GraphicDiffuseColor=[0.4 0.4 0.4]  CylinderLength=5  CylinderLengthUnits=m  CylinderRadius=1.5  CylinderRadiusUnits=m  Density=1000  DensityUnits=kg/m^3  DoExposeReferenceFrame=on  GraphicEmissiveColor=[0.0 0.0 0.0 1.0]  ExportEntireGeometry=off  SerializedFrames=<Frames/>  MarkerShape=Sphere  MarkerSize=10  GraphicType=FromGeometry  InertiaType=CalculateFromGeometry  Mass=1  MassUnits=kg  MomentsOfInertia=[1 1 1]  MomentsOfInertiaUnits=kg*m^2  GraphicOpacity=1.0  ProductsOfInertia=[0 0 0]  ProductsOfInertiaUnits=kg*m^2  GraphicShininess=75  GraphicSpecularColor=[0.5 0.5 0.5 1.0]  GraphicVisPropType=SimpleVisualProperties
  Spatial Contact Force : sm_lib/Forces and Torques/Spatial Contact Force  CoefficientOfDynamicFriction=0.3  CoefficientOfStaticFriction=0.5  NormalDamping=1e3  NormalDampingUnits=N/(m/s)  NormalStiffness=kBP  NormalStiffnessUnits=N/m  FrictionalCriticalVelocity=1e-3  FrictionalCriticalVelocityUnits=m/s  ZeroCrossDetectContactStartAndEnd=off  SenseFrictionalForceMagnitude=on  SenseNormalForceMagnitude=on  SenseSeparationDistance=on  NormalTransitionRegionWidth=0.05  NormalTransitionRegionWidthUnits=m  FrictionType=SmoothStickSlip
  Spatial Contact Force1 : sm_lib/Forces and Torques/Spatial Contact Force  CoefficientOfDynamicFriction=0.3  CoefficientOfStaticFriction=0.5  NormalDamping=1e3  NormalDampingUnits=N/(m/s)  NormalStiffness=kBP  NormalStiffnessUnits=N/m  FrictionalCriticalVelocity=1e-3  FrictionalCriticalVelocityUnits=m/s  ZeroCrossDetectContactStartAndEnd=off  SenseFrictionalForceMagnitude=on  SenseNormalForceMagnitude=on  SenseSeparationDistance=on  NormalTransitionRegionWidth=0.05  NormalTransitionRegionWidthUnits=m  FrictionType=SmoothStickSlip
  Spatial Contact Force2 : sm_lib/Forces and Torques/Spatial Contact Force  CoefficientOfDynamicFriction=0.3  CoefficientOfStaticFriction=0.5  NormalDamping=1e3  NormalDampingUnits=N/(m/s)  NormalStiffness=kBP  NormalStiffnessUnits=N/m  FrictionalCriticalVelocity=1e-3  FrictionalCriticalVelocityUnits=m/s  ZeroCrossDetectContactStartAndEnd=off  SenseFrictionalForceMagnitude=on  SenseNormalForceMagnitude=on  SenseSeparationDistance=on  NormalTransitionRegionWidth=0.05  NormalTransitionRegionWidthUnits=m  FrictionType=SmoothStickSlip
  Spherical Solid : sm_lib/Body Elements/Spherical Solid  GraphicAmbientColor=[0.15 0.15 0.15 1.0]  BasedOnType=Density  CenterOfMass=[0 0 0]  CenterOfMassUnits=m  GraphicDiffuseColor=[0.5 0.5 0.5]  Density=1000  DensityUnits=kg/m^3  DoExposeReferenceFrame=on  GraphicEmissiveColor=[0.0 0.0 0.0 1.0]  ExportEntireGeometry=on  SerializedExposedGeometries=<ExposedGeometries><ExposedGeometry><RawGeometryId>entire</RawGeometryId><ExposedGeometryId>G</ExposedGeometryId></ExposedGeometry></ExposedGeometries>  SerializedFrames=<Frames/>  MarkerShape=Sphere  MarkerSize=10  GraphicType=FromGeometry  InertiaType=CalculateFromGeometry  Mass=1  MassUnits=kg  MomentsOfInertia=[1 1 1]  MomentsOfInertiaUnits=kg*m^2  GraphicOpacity=1.0  ProductsOfInertia=[0 0 0]  ProductsOfInertiaUnits=kg*m^2  GraphicShininess=75  GraphicSpecularColor=[0.5 0.5 0.5 1.0]  SphereRadius=0.12  SphereRadiusUnits=m  GraphicVisPropType=SimpleVisualProperties
  Spherical Solid1 : sm_lib/Body Elements/Spherical Solid  GraphicAmbientColor=[0.15 0.15 0.15 1.0]  BasedOnType=Density  CenterOfMass=[0 0 0]  CenterOfMassUnits=m  GraphicDiffuseColor=[0.5 0.5 0.5]  Density=1000  DensityUnits=kg/m^3  DoExposeReferenceFrame=on  GraphicEmissiveColor=[0.0 0.0 0.0 1.0]  ExportEntireGeometry=on  SerializedExposedGeometries=<ExposedGeometries><ExposedGeometry><RawGeometryId>entire</RawGeometryId><ExposedGeometryId>G</ExposedGeometryId></ExposedGeometry></ExposedGeometries>  SerializedFrames=<Frames/>  MarkerShape=Sphere  MarkerSize=10  GraphicType=FromGeometry  InertiaType=CalculateFromGeometry  Mass=1  MassUnits=kg  MomentsOfInertia=[1 1 1]  MomentsOfInertiaUnits=kg*m^2  GraphicOpacity=1.0  ProductsOfInertia=[0 0 0]  ProductsOfInertiaUnits=kg*m^2  GraphicShininess=75  GraphicSpecularColor=[0.5 0.5 0.5 1.0]  SphereRadius=0.12  SphereRadiusUnits=m  GraphicVisPropType=SimpleVisualProperties
  Spherical Solid2 : sm_lib/Body Elements/Spherical Solid  GraphicAmbientColor=[0.15 0.15 0.15 1.0]  BasedOnType=Density  CenterOfMass=[0 0 0]  CenterOfMassUnits=m  GraphicDiffuseColor=[0.5 0.5 0.5]  Density=1000  DensityUnits=kg/m^3  DoExposeReferenceFrame=on  GraphicEmissiveColor=[0.0 0.0 0.0 1.0]  ExportEntireGeometry=on  SerializedExposedGeometries=<ExposedGeometries><ExposedGeometry><RawGeometryId>entire</RawGeometryId><ExposedGeometryId>G</ExposedGeometryId></ExposedGeometry></ExposedGeometries>  SerializedFrames=<Frames/>  MarkerShape=Sphere  MarkerSize=10  GraphicType=FromGeometry  InertiaType=CalculateFromGeometry  Mass=1  MassUnits=kg  MomentsOfInertia=[1 1 1]  MomentsOfInertiaUnits=kg*m^2  GraphicOpacity=1.0  ProductsOfInertia=[0 0 0]  ProductsOfInertiaUnits=kg*m^2  GraphicShininess=75  GraphicSpecularColor=[0.5 0.5 0.5 1.0]  SphereRadius=0.12  SphereRadiusUnits=m  GraphicVisPropType=SimpleVisualProperties
  To Workspace1 : ToWorkspace  VariableName=ds2  SampleTime=ts_control
  To Workspace2 : ToWorkspace  VariableName=ds1  SampleTime=ts_control
  To Workspace3 : ToWorkspace  VariableName=fn1  SampleTime=ts_control
  To Workspace4 : ToWorkspace  VariableName=fn2  SampleTime=ts_control
  To Workspace5 : ToWorkspace  VariableName=ds3  SampleTime=ts_control
  To Workspace6 : ToWorkspace  VariableName=fn3  SampleTime=ts_control
  To Workspace7 : ToWorkspace  VariableName=ffric1  SampleTime=ts_control
  To Workspace8 : ToWorkspace  VariableName=ffric2  SampleTime=ts_control
  To Workspace9 : ToWorkspace  VariableName=ffric3  SampleTime=ts_control
  World Frame : PMIOPort  Side=Left
  Conn2 : PMIOPort  Port=2  Side=Right
  BP1 Con : PMIOPort  Port=3  Side=Right
  BP2 Con : PMIOPort  Port=4  Side=Right
  BP3 Con : PMIOPort  Port=5  Side=Right
  wires:
  PS-Simulink Converter1/1 -> To Workspace5/1
  PS-Simulink Converter4/1 -> To Workspace1/1
  PS-Simulink Converter7/1 -> To Workspace2/1
  PS-Simulink Converter8/1 -> To Workspace3/1
  PS-Simulink Converter5/1 -> To Workspace4/1
  PS-Simulink Converter2/1 -> To Workspace6/1
  PS-Simulink Converter9/1 -> To Workspace7/1
  PS-Simulink Converter6/1 -> To Workspace8/1
  PS-Simulink Converter3/1 -> To Workspace9/1
  connections:
  Conn2/RConn1 -- Rigid Transform/RConn1
  Rigid Transform/LConn1 -- Rigid Transform3/LConn1 -- Rigid Transform2/LConn1 -- Rigid Transform1/LConn1 -- Solid/RConn1 -- World Frame/RConn1
  BP1/RConn1 -- Rigid Transform1/RConn1 -- Rigid Transform4/LConn1
  BP2/RConn1 -- Rigid Transform2/RConn1 -- Rigid Transform5/LConn1
  BP3/RConn1 -- Rigid Transform3/RConn1 -- Rigid Transform6/LConn1
  Spherical Solid2/RConn1 -- Rigid Transform4/RConn1
  Spherical Solid1/RConn1 -- Rigid Transform5/RConn1
  Spherical Solid/RConn1 -- Rigid Transform6/RConn1
  Spatial Contact Force2/LConn1 -- Spherical Solid/LConn1
  Spatial Contact Force1/LConn1 -- Spherical Solid1/LConn1
  Spatial Contact Force/LConn1 -- Spherical Solid2/LConn1
  BP1 Con/RConn1 -- Spatial Contact Force/RConn1
  BP3 Con/RConn1 -- Spatial Contact Force2/RConn1
  BP2 Con/RConn1 -- Spatial Contact Force1/RConn1
  PS-Simulink Converter1/LConn1 -- Spatial Contact Force2/RConn2
  PS-Simulink Converter2/LConn1 -- Spatial Contact Force2/RConn3
  PS-Simulink Converter3/LConn1 -- Spatial Contact Force2/RConn4
  PS-Simulink Converter4/LConn1 -- Spatial Contact Force1/RConn2
  PS-Simulink Converter5/LConn1 -- Spatial Contact Force1/RConn3
  PS-Simulink Converter6/LConn1 -- Spatial Contact Force1/RConn4
  PS-Simulink Converter7/LConn1 -- Spatial Contact Force/RConn2
  PS-Simulink Converter8/LConn1 -- Spatial Contact Force/RConn3
  PS-Simulink Converter9/LConn1 -- Spatial Contact Force/RConn4

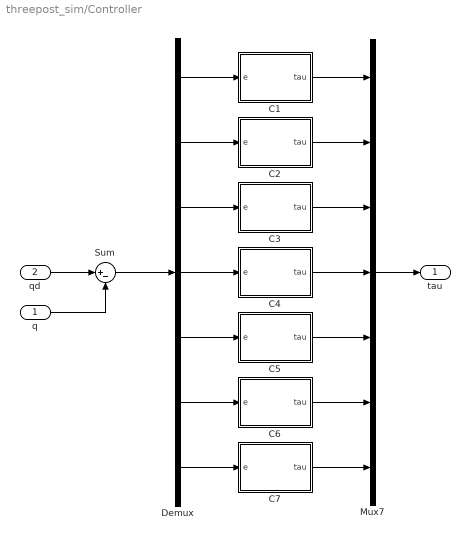
== system threepost_sim/Controller ==
  q : Inport
  qd : Inport  Port=2
  C1 : Subsystem
  C2 : Subsystem
  C3 : Subsystem
  C4 : Subsystem
  C5 : Subsystem
  C6 : Subsystem
  C7 : Subsystem
  Demux : Demux  Outputs=7
  Mux7 : Mux  Inputs=7
  Sum : Sum  Inputs=|+-
  tau : Outport
  wires:
  Mux7/1 -> tau/1
  C1/1(tau) -> Mux7/1
  C2/1(tau) -> Mux7/2
  C3/1(tau) -> Mux7/3
  C4/1(tau) -> Mux7/4
  C5/1(tau) -> Mux7/5
  C6/1(tau) -> Mux7/6
  C7/1(tau) -> Mux7/7
  Demux/1 -> C1/1(e)
  Demux/2 -> C2/1(e)
  Demux/3 -> C3/1(e)
  Demux/4 -> C4/1(e)
  Demux/5 -> C5/1(e)
  Demux/6 -> C6/1(e)
  Demux/7 -> C7/1(e)
  Sum/1 -> Demux/1
  q/1 -> Sum/2
  qd/1 -> Sum/1

== system threepost_sim/Forward Kinematics ==
  q : Inport
  Forward Kinematics : MATLAB Function  TreatAsAtomicUnit=on
  p : Outport
  R : Outport  Port=2
  wires:
  q/1 -> Forward Kinematics/1(q)
  Forward Kinematics/2(p) -> p/1
  Forward Kinematics/1(R) -> R/1
